simulink model "going"  (Simulink 7.5)
settings: Solver=ode3  StartTime=0.0  StopTime=10  FixedStep=.05  RelTol=1e-3
undefined symbols (not defined in the file or in its folder): CR, serial
libraries: instrumentlib x5, simulink x1, realtime_pacer_lib x1
settings Model: Creator=TCA  LastModifiedBy=bujiie
settings OptimizationCC: InitFltsAndDblsToZero=on
settings DebuggingCC: StrictBusMsg=Warning

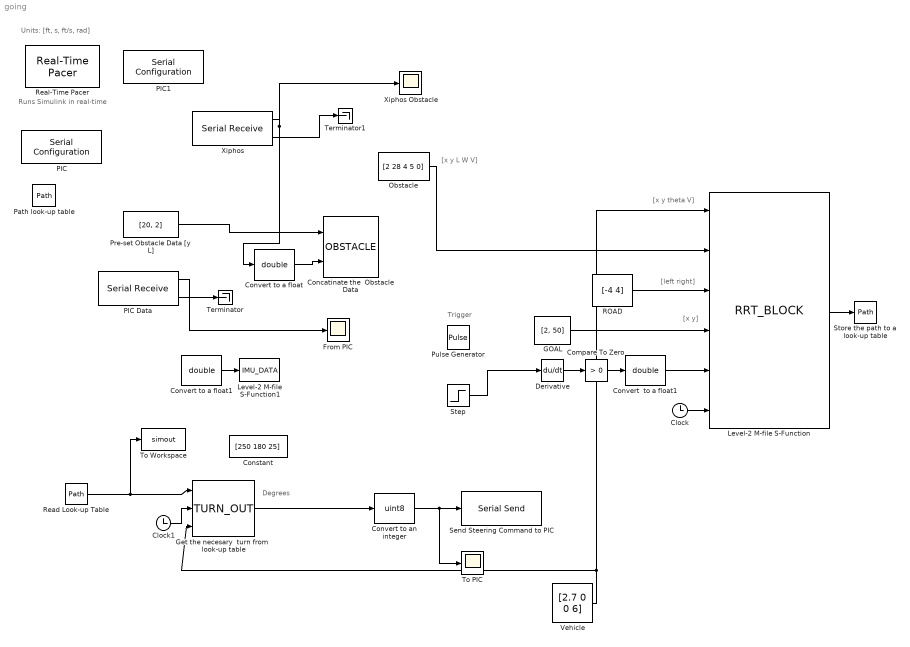
== system going ==
  note: [x y theta V]
  note: [x y L W V]
  note: [left right]
  note: [x y]
  note: Units: [ft, s, ft/s, rad]
  note: Trigger
  note: Degrees
  note: Runs Simulink
      |  in real-time
  Clock : Clock
      settings: Decimation=10
  Clock1 : Clock
      settings: Decimation=10
  Compare To Zero : simulink/Logic and Bit Operations/Compare To Zero  SystemSampleTime=-1  relop=>  LogicOutDataTypeMode=uint8  ZeroCross=off
  Concatinate the  Obstacle Data : M-S-Function  FunctionName=OBSTACLE  Parameters=2
  Constant : Constant  Value=[250 180 25]  OutDataType=fixdt(1, 16)  OutScaling=2^0
  Convert to a float : DataTypeConversion  OutDataTypeMode=double  OutDataTypeStr=double  SaturateOnIntegerOverflow=on  RndMeth=Zero
  Convert to a float1 : DataTypeConversion  OutDataTypeMode=double  OutDataTypeStr=double  SaturateOnIntegerOverflow=on  RndMeth=Zero
  Convert  to a float1 : DataTypeConversion  OutDataTypeMode=double  OutDataTypeStr=double  SaturateOnIntegerOverflow=on  RndMeth=Zero
  Convert to an integer : DataTypeConversion  OutDataTypeMode=uint8  OutDataTypeStr=uint8  SampleTime=.05  SaturateOnIntegerOverflow=on  RndMeth=Zero
  Derivative : Derivative
  From PIC : Scope
      settings: TimeRange=10  YMin=-1  YMax=1
  GOAL : Constant  Value=[2, 50]  VectorParams1D=off
  Get the necesary  turn from  look-up table : M-S-Function  FunctionName=TURN_OUT  Parameters=3
  Level-2 M-file S-Function : M-S-Function  FunctionName=RRT_BLOCK  Parameters=6
  Level-2 M-file S-Function1 : M-S-Function  FunctionName=IMU_DATA  Parameters=1
  Obstacle : Constant  Value=[2 28 4 5 0]  VectorParams1D=off
  PIC : instrumentlib/Serial Configuration  Priority=-200000  DialogController=instrumentcreatedialog  DialogControllerArgs=DataTag0  ComPortMenu=COM3  ComPort=COM3  ObjConstructor=serial('COM3');  BaudRate=115200  DataBits=8  Parity=none  StopBits=1  FlowControl=none  Timeout=10  ByteOrder=LittleEndian
  PIC Data : instrumentlib/Serial Receive  DialogController=instrumentcreatedialog  DialogControllerArgs=DataTag1  ComPortMenu=COM3  ComPort=COM3  ObjConstructor=serial('COM3');  Terminator=CR ('\r')  DataSize="[1  1]"  DataType=uint8  EnableBlockingMode=off  ActionDataUnavailable=Output last received value  CustomValue=0  SampleTime=0.05
  PIC1 : instrumentlib/Serial Configuration  Priority=-200000  DialogController=instrumentcreatedialog  DialogControllerArgs=DataTag2  ComPortMenu=COM5  ComPort=COM5  ObjConstructor=serial('COM5');  BaudRate=9600  DataBits=8  Parity=none  StopBits=1  FlowControl=none  Timeout=10  ByteOrder=LittleEndian
  Path look-up table : DataStoreMemory  DataStoreName=Path  ReadBeforeWriteMsg=warning  WriteAfterWriteMsg=warning  WriteAfterReadMsg=warning  InitialValue=zeros(50, 6)  VectorParams1D=off
  Pre-set Obstacle Data [y L] : Constant  Value=[20, 2]  OutDataType=fixdt(1, 16)  OutScaling=2^0  SampleTime=.05
  Pulse Generator : DiscretePulseGenerator  PulseType=Time based  Amplitude=1  Period=1  PulseWidth=5  PhaseDelay=0  SampleTime=1
  ROAD : Constant  Value=[-4 4]  VectorParams1D=off
  Read Look-up Table : DataStoreRead  DataStoreName=Path  SampleTime=0
  Real-Time Pacer : realtime_pacer_lib/Real-Time Pacer  simTimePerRealTime=1
  Send Steering Command to PIC : instrumentlib/Serial Send  DialogController=instrumentcreatedialog  DialogControllerArgs=DataTag3  ComPortMenu=COM3  ComPort=COM3  ObjConstructor=serial('COM3');  Terminator=<none>  EnableBlockingMode=off
  Step : Step  Time=1.5  SampleTime=0
  Store the path to a look-up table : DataStoreWrite  DataStoreName=Path  SampleTime=-1
  Terminator : Terminator
  Terminator1 : Terminator
  To PIC : Scope
      settings: TimeRange=10  YMin=120  YMax=250  SaveName=ScopeData4
  To Workspace : ToWorkspace  VariableName=simout  SampleTime=-1  SaveFormat=Array
  Vehicle : Constant  Value=[2.7 0 0 6]  VectorParams1D=off
  Xiphos : instrumentlib/Serial Receive  DialogController=instrumentcreatedialog  DialogControllerArgs=DataTag4  ComPortMenu=COM5  ComPort=COM5  ObjConstructor=serial('COM5');  Terminator=CR ('\r')  DataSize="[1  3]"  DataType=int8  EnableBlockingMode=off  ActionDataUnavailable=Output last received value  CustomValue=0  SampleTime=0.05
  Xiphos Obstacle : Scope
      settings: TimeRange=10  YMax=25
  wires:
  PIC Data/2 -> Terminator/1
  Vehicle/1 -> Level-2 M-file S-Function/1, Get the necesary  turn from  look-up table/3
  ROAD/1 -> Level-2 M-file S-Function/3
  GOAL/1 -> Level-2 M-file S-Function/4
  Read Look-up Table/1 -> Get the necesary  turn from  look-up table/1, To Workspace/1
  Compare To Zero/1 -> Convert  to a float1/1
  Level-2 M-file S-Function/1 -> Store the path to a look-up table/1
  Convert  to a float1/1 -> Level-2 M-file S-Function/5
  Derivative/1 -> Compare To Zero/1
  Clock/1 -> Level-2 M-file S-Function/6
  Clock1/1 -> Get the necesary  turn from  look-up table/2
  Step/1 -> Derivative/1
  Convert to an integer/1 -> Send Steering Command to PIC/1, To PIC/1
  Pre-set Obstacle Data [y L]/1 -> Concatinate the  Obstacle Data/1
  Convert to a float/1 -> Concatinate the  Obstacle Data/2
  Get the necesary  turn from  look-up table/1 -> Convert to an integer/1
  Convert to a float1/1 -> Level-2 M-file S-Function1/1
  PIC Data/1 -> From PIC/1
  Xiphos/1 -> Convert to a float/1, Xiphos Obstacle/1
  Xiphos/2 -> Terminator1/1
  Obstacle/1 -> Level-2 M-file S-Function/2
